simulink model "Temp"  (Simulink 7.7)
settings: Solver=ode45  StartTime=0.0  StopTime=10  RelTol=1e-3
PreLoadFcn:
  | EbNo = 16; Errors = 188; Bits = 1e8; M = 256; N = 64; Ts = (1/22050); constellation; InnerInterleaverBitTable
undefined symbols (not defined in the file or in its folder): gray, rsgenpoly
libraries: commutil2 x4, commblkintrlv2 x4, vipsnks x3, commblkcod2 x2, commcnvintrlv2 x2, commsink2 x2, commcnvcod2 x2, dspsigops x2, dspxfrm3 x2, commdigbbndam3 x2, dspsnks4 x1, dspmtrx3 x1
settings Model: Creator=katsikas  LastModifiedBy=katsikas
settings SimEventsCC: propDiagAttribOutput=1  propDiagFcnCallOutput=1  propDiagStatOutput=0

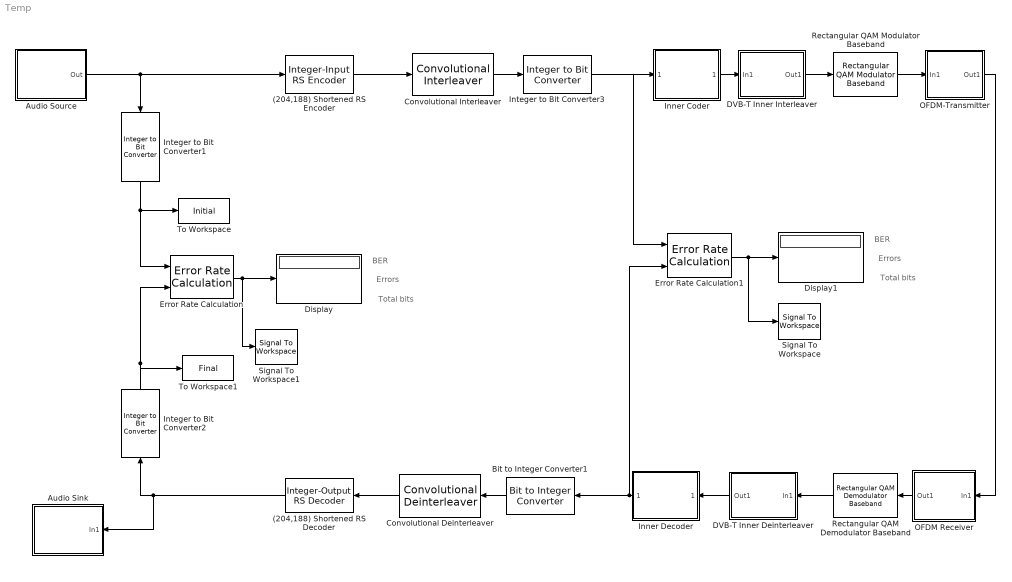
== system Temp ==
  note: BER
  note: Total bits
  note: Errors
  note: BER
  note: Total bits
  note: Errors
  (204,188) Shortened RS Decoder : commblkcod2/Integer-Output RS Decoder  n=204  k=188  specPrimPoly=off  prPoly=[1 0 1 1]  specGenPoly=off  genPoly=rsgenpoly(7,3)  specPuncture=off  punctVec=[ones(2,1); zeros(2,1)]  specErasurePort=off  showNumErr=off
  (204,188) Shortened RS Encoder : commblkcod2/Integer-Input RS Encoder  n=204  k=188  specPrimPoly=off  prPoly=[1 0 1 1]  specGenPoly=off  genPoly=rsgenpoly(7,3)  specPuncture=off  punctVec=[ones(2,1); zeros(2,1)]
  Audio Sink : Subsystem
  Audio Source : Subsystem
  Bit to Integer Converter1 : commutil2/Bit to Integer Converter  nbits=log2(M)  bitOrder=MSB first  signedOutputValues=Unsigned  outDtype=uint8  outDtypeSigned=Inherit via internal rule
  Convolutional Deinterleaver : commcnvintrlv2/Convolutional Deinterleaver  SystemSampleTime=-1  N=12  B=17  ic=0
  Convolutional Interleaver : commcnvintrlv2/Convolutional Interleaver  SystemSampleTime=-1  N=12  B=17  ic=0
  DVB-T Inner Deinterleaver : Subsystem  mask(DVB-T Inner Deinterleaver){}
      mask init:
      | fullILVec = [(1:126) ...
      |  (rem([0:125]+63,126) +1 + 126     ) ...
      |  (rem([0:125]+105,126)+1 + (2*126) ) ...
      |  (rem([0:125]+42,126) +1 + (3*126) ) ...
      |  (rem([0:125]+21,126) +1 + (4*126) ) ...
      |  (rem([0:125]+84,126) +1 + (5*126) )];
      mask Display: disp('DVB-T\nInner\nDeinterleaver')
  DVB-T Inner Interleaver : Subsystem  mask(DVB-T Inner Interleaver){}
      mask init: same as Temp/DVB-T Inner Deinterleaver
      mask Display: disp('DVB-T\nInner\nInterleaver')
  Display : Display
  Display1 : Display
  Error Rate Calculation : commsink2/Error Rate Calculation  N=188*17*8  st_delay=0  cp_mode=Entire frame  subframe=[]  PMode=Port  WsName=ErrorVec  RsMode2=off  stop=off  numErr=Errors  maxBits=Bits
  Error Rate Calculation1 : commsink2/Error Rate Calculation  N=1632*6  st_delay=0  cp_mode=Entire frame  subframe=[]  PMode=Port  WsName=ErrorVec  RsMode2=off  stop=off  numErr=100  maxBits=1e8
  Inner Coder : Subsystem
      mask Display: disp('Rate 3/4\nPunctured\nConvolutional\nCode');
  Inner Decoder : Subsystem
      mask Display: disp('Viterbi\nDecoder')
  Integer to Bit Converter1 : commutil2/Integer to Bit Converter  nbits=8  signedInputValues=Unsigned  bitOrder=MSB first  outDtype=boolean
  Integer to Bit Converter2 : commutil2/Integer to Bit Converter  nbits=8  signedInputValues=Unsigned  bitOrder=MSB first  outDtype=boolean
  Integer to Bit Converter3 : commutil2/Integer to Bit Converter  nbits=log2(M)  signedInputValues=Unsigned  bitOrder=MSB first  outDtype=boolean
  OFDM Receiver : Subsystem
  OFDM-Transmitter : Subsystem
  Rectangular QAM Demodulator Baseband : commdigbbndam3/Rectangular QAM Demodulator Baseband  M=N  PowType=Average Power  MinDist=2  AvgPow=1  PeakPow=1  Ph=0  Dec=User-defined  Mapping=map_constellation  OutType=Bit  DecType=Hard decision  VarSource=Dialog  Variance=1  outDtype1=boolean  outDtype2=Inherit via internal rule  derotateFactorWordLen=16  denormFactorWordLen=16  prodOutWordLen=32  prodOutRoundingMode=Floor  prodOutOverflowMode=Wrap  sumWordLen=32
  Rectangular QAM Modulator Baseband : commdigbbndam3/Rectangular QAM Modulator Baseband  M=N  InType=Bit  Enc=User-defined  Mapping=map_constellation  PowType=Average Power  MinDist=2  AvgPow=1  PeakPow=1  Ph=0  outDtype=double  outWordLen=16  outUDDataType=sfix(16)  outFracLenMode=Best precision  outFracLen=15
  Signal To Workspace : SignalToWorkspace  VariableName=BER1  SaveFormat=Array  Save2DMode=2-D array (concatenate along first dimension)
      settings: CopyFcn=dspblkcopystw(gcbh);
  Signal To Workspace1 : SignalToWorkspace  VariableName=BER  SaveFormat=Array  Save2DMode=2-D array (concatenate along first dimension)
      settings: CopyFcn=dspblkcopystw(gcbh);  MaxDataPoints=1
  To Workspace : ToWorkspace  VariableName=Initial  SampleTime=-1  SaveFormat=Array
  To Workspace1 : ToWorkspace  VariableName=Final  SampleTime=-1  SaveFormat=Array
  wires:
  Error Rate Calculation/1 -> Display/1, Signal To Workspace1/1
  Integer to Bit Converter2/1 -> Error Rate Calculation/2, To Workspace1/1
  (204,188) Shortened RS Decoder/1 -> Integer to Bit Converter2/1, Audio Sink/1(In1)
  Rectangular QAM Modulator Baseband/1 -> OFDM-Transmitter/1(In1)
  Convolutional Interleaver/1 -> Integer to Bit Converter3/1
  Convolutional Deinterleaver/1 -> (204,188) Shortened RS Decoder/1
  (204,188) Shortened RS Encoder/1 -> Convolutional Interleaver/1
  Error Rate Calculation1/1 -> Display1/1, Signal To Workspace/1
  Integer to Bit Converter3/1 -> Inner Coder/1(Uncoded symbols), Error Rate Calculation1/1
  Rectangular QAM Demodulator Baseband/1 -> DVB-T Inner Deinterleaver/1(In1)
  Bit to Integer Converter1/1 -> Convolutional Deinterleaver/1
  Inner Coder/1(Coded bits) -> DVB-T Inner Interleaver/1(In1)
  Inner Decoder/1(Decoded symbols) -> Bit to Integer Converter1/1, Error Rate Calculation1/2
  DVB-T Inner Interleaver/1(Out1) -> Rectangular QAM Modulator Baseband/1
  DVB-T Inner Deinterleaver/1(Out1) -> Inner Decoder/1(Received bits)
  OFDM Receiver/1(Out1) -> Rectangular QAM Demodulator Baseband/1
  OFDM-Transmitter/1(Out1) -> OFDM Receiver/1(In1)
  Integer to Bit Converter1/1 -> Error Rate Calculation/1, To Workspace/1
  Audio Source/1(Out) -> Integer to Bit Converter1/1, (204,188) Shortened RS Encoder/1

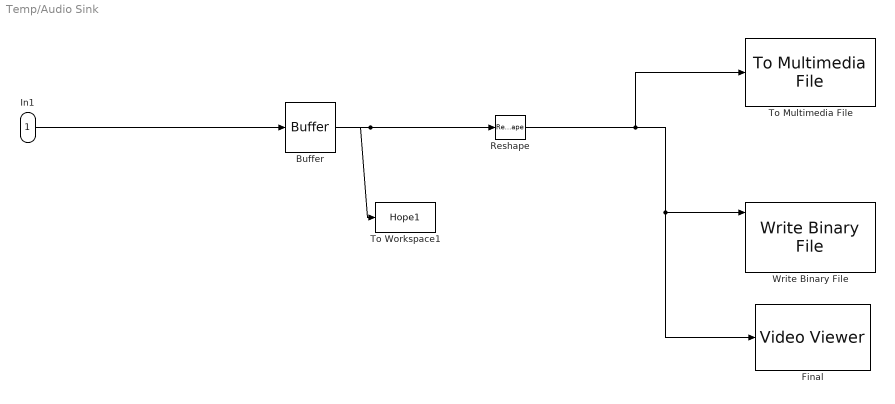
== system Temp/Audio Sink ==
  In1 : Inport
  Buffer : Buffer  N=19200  TreatMby1Signals=One channel
  Final : vipsnks/Video Viewer  inputType=Obsolete7b  imagePorts=One multidimensional signal  useColorMap=off  colormapValue=gray(256)  specRange=off  minInputVal=0  maxInputVal=255  FigPos=[463 935 458 411]  AxisZoom=on  trueSizedOnce=on  OpenAtMdlStart=on
  Reshape : Reshape  OutputDimensionality=Customize  OutputDimensions=[160,120]
  To Multimedia File : dspsnks4/To Multimedia File  outputFilename=output.avi  streamSelection=Video only  videoCompressor=None (uncompressed)  audioCompressor=None (uncompressed)  imagePorts=One multidimensional signal  fileType=AVI  audioDatatype=Determine from input data type  fourcc=RGB
  To Workspace1 : ToWorkspace  VariableName=Hope1  SampleTime=-1  SaveFormat=Array
  Write Binary File : vipsnks/Write Binary File  FileName=output.bin  VideoFormat=Four character codes  FOURCC=I420  BitStreamFormat=Planar  NumInputs=3  ComponentOrder=[1 2 3]  Interlaced=off  LineOrdering=Top line first  InheritBits=on  Component1=Y'  Component2=Cb  Component3=Cr  Component4=Alpha  Bits1=8  Bits2=8  Bits3=8  Bits4=0  SignedInput=off  FileEndian=Little endian
  wires:
  Reshape/1 -> Final/1, Write Binary File/1, To Multimedia File/1
  Buffer/1 -> Reshape/1, To Workspace1/1
  In1/1 -> Buffer/1

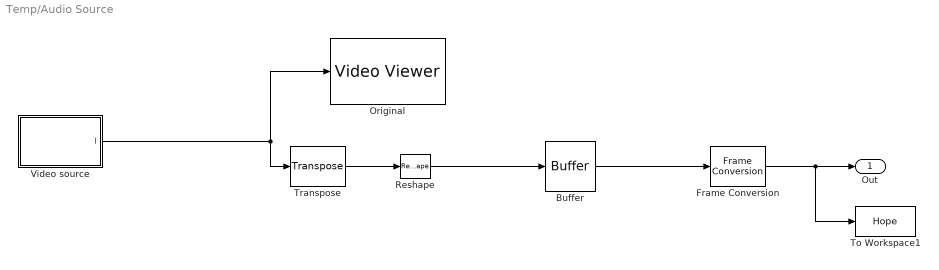
== system Temp/Audio Source ==
  Buffer : Buffer  N=188  TreatMby1Signals=One channel
  Frame Conversion : FrameConversion
  Original : vipsnks/Video Viewer  inputType=Obsolete7b  imagePorts=One multidimensional signal  useColorMap=off  colormapValue=gray(256)  specRange=off  minInputVal=0  maxInputVal=255  FigPos=[54 877 458 411]  AxisZoom=on  trueSizedOnce=on  OpenAtMdlStart=on
  Reshape : Reshape
  To Workspace1 : ToWorkspace  VariableName=Hope  SampleTime=-1  SaveFormat=Array
  Transpose : dspmtrx3/Transpose  SystemSampleTime=-1  Hermitian=off  overflowFlag=off
  Video source : Subsystem
  Out : Outport
  wires:
  Reshape/1 -> Buffer/1
  Video source/1(I) -> Original/1, Transpose/1
  Transpose/1 -> Reshape/1
  Buffer/1 -> Frame Conversion/1
  Frame Conversion/1 -> Out/1, To Workspace1/1

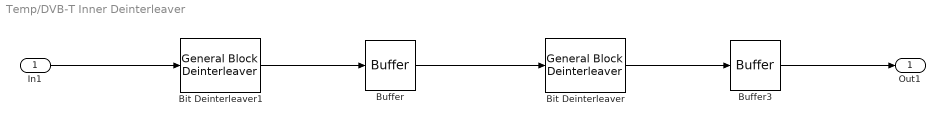
== system Temp/DVB-T Inner Deinterleaver ==
  In1 : Inport
  Bit Deinterleaver : commblkintrlv2/General Block Deinterleaver  elements=BitInterleaverTable
  Bit Deinterleaver1 : commblkintrlv2/General Block Deinterleaver  elements=SymbolInterleaverTable
  Buffer : Buffer  N=756  TreatMby1Signals=One channel
  Buffer3 : Buffer  N=2176  TreatMby1Signals=One channel
  Out1 : Outport
  wires:
  In1/1 -> Bit Deinterleaver1/1
  Buffer3/1 -> Out1/1
  Buffer/1 -> Bit Deinterleaver/1
  Bit Deinterleaver/1 -> Buffer3/1
  Bit Deinterleaver1/1 -> Buffer/1

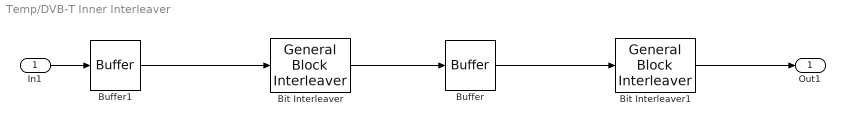
== system Temp/DVB-T Inner Interleaver ==
  In1 : Inport
  Bit Interleaver : commblkintrlv2/General Block Interleaver  elements=BitInterleaverTable
  Bit Interleaver1 : commblkintrlv2/General Block Interleaver  elements=SymbolInterleaverTable
  Buffer : Buffer  N=9072  TreatMby1Signals=One channel
  Buffer1 : Buffer  N=756  TreatMby1Signals=One channel
  Out1 : Outport
  wires:
  In1/1 -> Buffer1/1
  Buffer/1 -> Bit Interleaver1/1
  Buffer1/1 -> Bit Interleaver/1
  Bit Interleaver/1 -> Buffer/1
  Bit Interleaver1/1 -> Out1/1

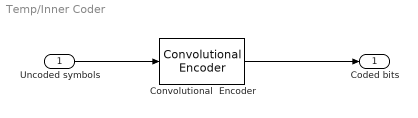
== system Temp/Inner Coder ==
  Uncoded symbols : Inport
  Convolutional  Encoder : commcnvcod2/Convolutional Encoder  trellis=poly2trellis(7, [171 133])  opMode=Continuous  DelayedResetAction=off  hasIniStPort=off  hasFinStPort=off  usePuncVector=on  punctureVector=[1 1 0 1 1 0]'  reset=Unused parameter value
  Coded bits : Outport
  wires:
  Convolutional  Encoder/1 -> Coded bits/1
  Uncoded symbols/1 -> Convolutional  Encoder/1

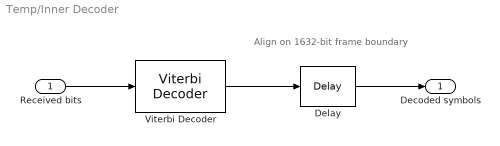
== system Temp/Inner Decoder ==
  note: Align on 1632-bit
      | frame boundary
  Received bits : Inport
  Delay : dspsigops/Delay  InputProcessing=Columns as channels (frame based)  dly_unit=Samples  delay=584+69  ic_detail=off  dif_ic_for_ch=off  dif_ic_for_dly=off  ic=0  reset_popup=None
  Viterbi Decoder : commcnvcod2/Viterbi Decoder  trellis=poly2trellis(7, [171 133])  isPunctured=on  punctureVector=[1 1 0 1 1 0]'  erasures=off  dectype=Hard decision  runSigValErrCheck=off  nsdecb=4  smWordLength=16  tbdepth=136  opmode=Continuous  reset=off  outDataType=boolean
  Decoded symbols : Outport
  wires:
  Viterbi Decoder/1 -> Delay/1
  Received bits/1 -> Viterbi Decoder/1
  Delay/1 -> Decoded symbols/1

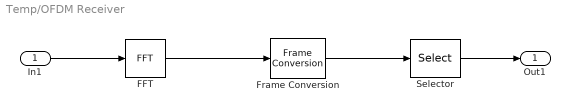
== system Temp/OFDM Receiver ==
  In1 : Inport
  FFT : dspxfrm3/FFT  CompMethod=Table lookup  TableOpt=NEW  TableOptActive=Speed  BitRevOrder=off  InheritFFTLength=on  FFTLength=64  RowConvenienceOn=on  SkipNorm=off  firstCoeffDataTypeStr=Inherit: Same word length as input  firstCoeffLastDataTypeStr=Inherit: Same word length as input  outputMin=[]  outputMax=[]  roundingMode=Floor  overflowMode=off
  Frame Conversion : FrameConversion
  Selector : Selector  NumberOfDimensions=2  InputPortWidth=3  IndexOptions=Index vector (dialog),Select all  Indices=[1:756 1293:2048],1  OutputSizes=1,1
  Out1 : Outport
  wires:
  FFT/1 -> Frame Conversion/1
  Frame Conversion/1 -> Selector/1
  In1/1 -> FFT/1
  Selector/1 -> Out1/1

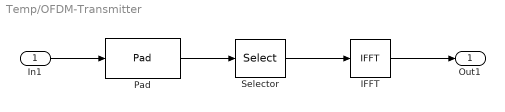
== system Temp/OFDM-Transmitter ==
  In1 : Inport
  IFFT : dspxfrm3/IFFT  CompMethod=Table lookup  TableOpt=NEW  TableOptActive=Speed  BitRevOrder=off  cs_in=off  SkipNorm=on  InheritFFTLength=on  FFTLength=64  mode=Complex  outSamplingMode=Frame based  RowConvenienceOn=on  firstCoeffDataTypeStr=Inherit: Same word length as input  firstCoeffLastDataTypeStr=Inherit: Same word length as input  outputMin=[]  outputMax=[]  roundingMode=Floor  overflowMode=off
  Pad : dspsigops/Pad  padAlong=Columns  dimsToPad=1  valSrc=Specify via dialog  padVal=0  spec=Output size  padNumOutRowsSpecMethod=User-specified  numOutRows=2048  padNumOutColsSpecMethod=User-specified  numOutCols=1  isVarDimsMode=off  padBeginning=0  padEnd=0  outSizeMode=User-specified  outSize=1  padSigAt=End  trunc_flag=None  roundingMode=Floor  overflowMode=off  truncOrWrapMode=Truncate  wrap_flag=None
  Selector : Selector  NumberOfDimensions=2  InputPortWidth=3  IndexOptions=Index vector (dialog),Select all  Indices=[1:756 1513:2048 757:1512],1  OutputSizes=1,1
  Out1 : Outport
  wires:
  Pad/1 -> Selector/1
  Selector/1 -> IFFT/1
  IFFT/1 -> Out1/1
  In1/1 -> Pad/1

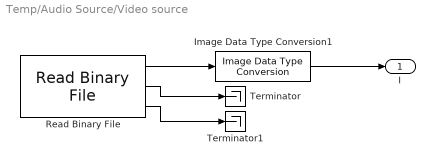
== system Temp/Audio Source/Video source ==
  Image Data Type Conversion1 : vipconversions/Image Data Type Conversion  outDT=uint8  isSigned=on  wordLen=16  numFracBits=0
  Read Binary File : vipsrcs/Read Binary File  FileName=vipmen.bin  loopOrNot=on  numLoops=inf  VideoFormat=Custom  FOURCC=I420  BitStreamFormat=Planar  NumOutputs=3  ComponentOrder=[1 2 3]  Interlaced=off  LineOrdering=Top line first  Ts=1/30  Component1=Y'  Component2=Cb  Component3=Cr  Component4=Alpha  Bits1=8  Bits2=8  Bits3=8  Bits4=8  Rows1=120  Rows2=60  Rows3=60  Rows4=288  Cols1=160  Cols2=80  Cols3=80  Cols4=352  YRows=288  YCols=352  SignedOutput=off  FileEndian=Little endian  OutputEOF=off
  Terminator : Terminator
  Terminator1 : Terminator
  I : Outport
  wires:
  Image Data Type Conversion1/1 -> I/1
  Read Binary File/1 -> Image Data Type Conversion1/1
  Read Binary File/2 -> Terminator/1
  Read Binary File/3 -> Terminator1/1
